simulink model "Mit"  (R2019a)
settings: Solver=VariableStepAuto  StartTime=0.0  StopTime=10.0  RelTol=1e-3
values from neighbouring files (symbols this model uses):
  B = 0.12    [Values.m]
  g = 100000000    [Values.m]
  J = 0.00004    (= 4e-05)    [Values.m]
  K = 0.235    [Values.m]
  L = 0.2    [Values.m]
  R = 5    [Values.m]
settings Model: Creator=MILAD ALMOHSEN  LastModifiedBy=MILAD ALMOHSEN

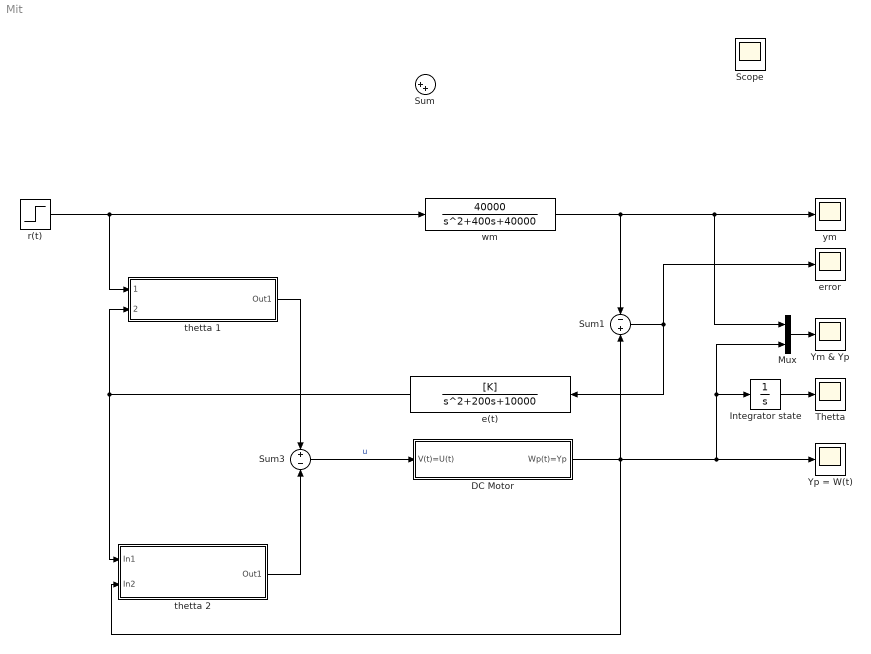
== system Mit ==
  DC Motor : Subsystem
  Integrator state : Integrator
  Mux : Mux  Inputs=2
  Scope : Scope
  Sum : Sum  Inputs=|++
  Sum1 : Sum  Inputs=-|+
  Sum3 : Sum  Inputs=+|-
  Thetta : Scope
  Ym & Yp : Scope
  Yp = W(t) : Scope
  "e(t) " : TransferFcn  Numerator=[K]  Denominator=[1 200 10000]
  error : Scope
  r(t) : Step  SampleTime=0
  thetta 1 : Subsystem
  thetta 2 : Subsystem
  wm : TransferFcn  Numerator=[40000]  Denominator=[1 400 40000]
  ym : Scope
  wires:
  r(t)/1 -> thetta 1/1(1), wm/1
  wm/1 -> Mux/1, ym/1, Sum1/1
  Sum1/1 -> error/1, "e(t) "/1
  DC Motor/1(Wp(t)=Yp) -> Integrator state/1, Mux/2, Yp = W(t)/1, thetta 2/2(In2), Sum1/2
  Integrator state/1 -> Thetta/1
  Sum3/1 -> DC Motor/1(V(t)=U(t))  "u"
  "e(t) "/1 -> thetta 1/2(2), thetta 2/1(In1)
  thetta 1/1(Out1) -> Sum3/1
  thetta 2/1(Out1) -> Sum3/2
  Mux/1 -> Ym & Yp/1

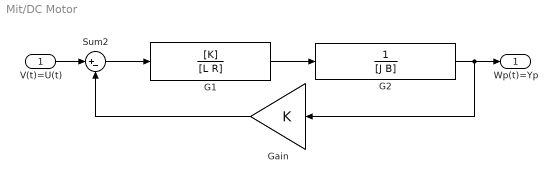
== system Mit/DC Motor ==
  V(t)=U(t) : Inport
  G1 : TransferFcn  Numerator=[K]  Denominator=[L R]
  G2 : TransferFcn  Denominator=[J B]
  Gain : Gain  Gain=K
  Sum2 : Sum  Inputs=|+-
  Wp(t)=Yp : Outport
  wires:
  G1/1 -> G2/1
  Sum2/1 -> G1/1
  G2/1 -> Wp(t)=Yp/1, Gain/1
  V(t)=U(t)/1 -> Sum2/1
  Gain/1 -> Sum2/2

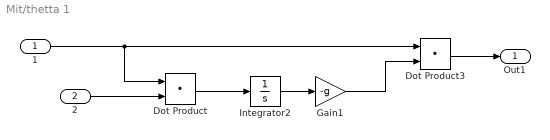
== system Mit/thetta 1 ==
  1 : Inport
  2 : Inport  Port=2
  Dot Product : DotProduct  InputSameDT=on  OutDataTypeStr=Inherit: Inherit via internal rule
  Dot Product3 : DotProduct  InputSameDT=on  OutDataTypeStr=Inherit: Inherit via internal rule
  Gain1 : Gain  Gain=-g
  Integrator2 : Integrator
  Out1 : Outport
  wires:
  2/1 -> Dot Product/2
  Gain1/1 -> Dot Product3/2
  Dot Product/1 -> Integrator2/1
  Integrator2/1 -> Gain1/1
  1/1 -> Dot Product/1, Dot Product3/1
  Dot Product3/1 -> Out1/1

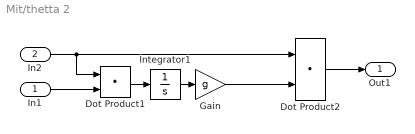
== system Mit/thetta 2 ==
  In1 : Inport
  In2 : Inport  Port=2
  Dot Product1 : DotProduct  InputSameDT=on  OutDataTypeStr=Inherit: Inherit via internal rule
  Dot Product2 : DotProduct  InputSameDT=on  OutDataTypeStr=Inherit: Inherit via internal rule
  Gain : Gain  Gain=g
  Integrator1 : Integrator
  Out1 : Outport
  wires:
  Integrator1/1 -> Gain/1
  In2/1 -> Dot Product1/1, Dot Product2/1
  Dot Product1/1 -> Integrator1/1
  In1/1 -> Dot Product1/2
  Gain/1 -> Dot Product2/2
  Dot Product2/1 -> Out1/1
